simulink model "insulinGlucoseSimHumanCtrl_Harness1"  (R2019a)
settings: Solver=ode3  StartTime=0  StopTime=500  RelTol=1e-3  EnableMultiTasking=on
settings Model: Creator=yangy  LastModifiedBy=yangy
settings SolverCC: MaxConsecutiveZCs=100
settings DataIOCC: LimitDataPoints=on  SaveFormat=Array  SignalLoggingSaveFormat=ModelDataLogs  ReturnWorkspaceOutputs=off
settings OptimizationCC: ExpressionDepthLimit=2147483647  LifeSpan=inf
settings DebuggingCC: UnderspecifiedInitializationDetection=Classic  MergeDetectMultiDrivingBlocksExec=none  FcnCallInpInsideContextMsg=warning  StateNameClashWarn=warning  SFUnexpectedBacktrackingDiag=warning  SFNoUnconditionalDefaultTransitionDiag=warning  SFExecutionAtInitializationDiag=none  ArithmeticOperatorsInVariantConditions=warning
settings HardwareCC: ProdBitPerPointer=32  ProdBitPerSizeT=32  ProdBitPerPtrDiffT=32  ProdLargestAtomicFloat=None  ProdIntDivRoundTo=Undefined  ProdEndianess=Unspecified  ProdWordSize=32  ProdHWDeviceType=32-bit Generic
settings ModelReferenceCC: PropagateSignalLabelsOutOfModel=off
settings SFSimCC: SimUseLocalCustomCode=off  SimParseCustomCode=off
settings RTWCC: RTWUseLocalCustomCode=off
settings CodeAppCC: StateflowObjectComments=on
settings GRTTargetCC: TargetLangStandard=C89/C90 (ANSI)  GeneratePreprocessorConditionals=Disable all  CombineOutputUpdateFcns=off  GRTInterface=on
settings ConfigComp: CovMetricSettings=dw  CovHtmlReporting=on  CovSaveCumulativeToWorkspaceVar=on  CovSaveSingleToWorkspaceVar=on  CovExternalEMLEnable=off

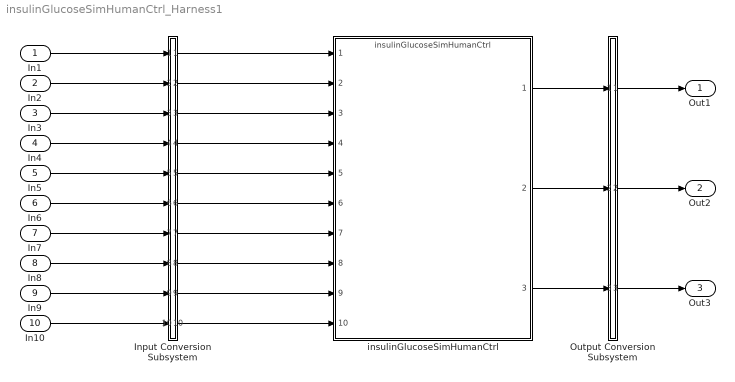
== system insulinGlucoseSimHumanCtrl_Harness1 ==
  In1 : Inport  OutDataTypeStr=double  PortDimensions=[1]  SampleTime=0
  In2 : Inport  Port=2  OutDataTypeStr=double  PortDimensions=[1]  SampleTime=0
  In3 : Inport  Port=3  OutDataTypeStr=double  PortDimensions=[1]  SampleTime=0
  In4 : Inport  Port=4  OutDataTypeStr=double  PortDimensions=[1]  SampleTime=0
  In5 : Inport  Port=5  OutDataTypeStr=double  PortDimensions=[1]  SampleTime=0
  In6 : Inport  Port=6  OutDataTypeStr=double  PortDimensions=[1]  SampleTime=0
  In7 : Inport  Port=7  OutDataTypeStr=double  PortDimensions=[1]  SampleTime=0
  In8 : Inport  Port=8  OutDataTypeStr=double  PortDimensions=[1]  SampleTime=0
  In9 : Inport  Port=9  OutDataTypeStr=double  PortDimensions=[1]  SampleTime=0
  In10 : Inport  Port=10  OutDataTypeStr=double  PortDimensions=[1]  SampleTime=0
  Input Conversion Subsystem : Subsystem  Tag=__SLT_ICS__  Description=|
      | Signal spec.
      | and routing
      settings: AttributesFormatString=%<Description>
  Output Conversion Subsystem : Subsystem  Tag=__SLT_OCS__  Description=|
      | Signal spec.
      | and routing
      settings: AttributesFormatString=%<Description>
  insulinGlucoseSimHumanCtrl : ModelReference  ModelNameDialog=insulinGlucoseSimHumanCtrl  SimulationMode=Normal  ModelReferenceVersion=1.334
  Out1 : Outport  OutDataTypeStr=double  PortDimensions=[1]
  Out2 : Outport  Port=2  OutDataTypeStr=double  PortDimensions=[1]
  Out3 : Outport  Port=3  OutDataTypeStr=double  PortDimensions=[1]
  wires:
  In1/1 -> Input Conversion Subsystem/1(Inport_1)
  In2/1 -> Input Conversion Subsystem/2(Inport_2)
  In3/1 -> Input Conversion Subsystem/3(Inport_3)
  In4/1 -> Input Conversion Subsystem/4(Inport_4)
  In5/1 -> Input Conversion Subsystem/5(Inport_5)
  In6/1 -> Input Conversion Subsystem/6(Inport_6)
  In7/1 -> Input Conversion Subsystem/7(Inport_7)
  In8/1 -> Input Conversion Subsystem/8(Inport_8)
  In9/1 -> Input Conversion Subsystem/9(Inport_9)
  In10/1 -> Input Conversion Subsystem/10(Inport_10)
  Output Conversion Subsystem/1(Outport_1) -> Out1/1
  Output Conversion Subsystem/2(Outport_2) -> Out2/1
  Output Conversion Subsystem/3(Outport_3) -> Out3/1
  Input Conversion Subsystem/1(Outport_1) -> insulinGlucoseSimHumanCtrl/1
  Input Conversion Subsystem/2(Outport_2) -> insulinGlucoseSimHumanCtrl/2
  Input Conversion Subsystem/3(Outport_3) -> insulinGlucoseSimHumanCtrl/3
  Input Conversion Subsystem/4(Outport_4) -> insulinGlucoseSimHumanCtrl/4
  Input Conversion Subsystem/5(Outport_5) -> insulinGlucoseSimHumanCtrl/5
  Input Conversion Subsystem/6(Outport_6) -> insulinGlucoseSimHumanCtrl/6
  Input Conversion Subsystem/7(Outport_7) -> insulinGlucoseSimHumanCtrl/7
  Input Conversion Subsystem/8(Outport_8) -> insulinGlucoseSimHumanCtrl/8
  Input Conversion Subsystem/9(Outport_9) -> insulinGlucoseSimHumanCtrl/9
  Input Conversion Subsystem/10(Outport_10) -> insulinGlucoseSimHumanCtrl/10
  insulinGlucoseSimHumanCtrl/1 -> Output Conversion Subsystem/1(Inport_1)
  insulinGlucoseSimHumanCtrl/2 -> Output Conversion Subsystem/2(Inport_2)
  insulinGlucoseSimHumanCtrl/3 -> Output Conversion Subsystem/3(Inport_3)

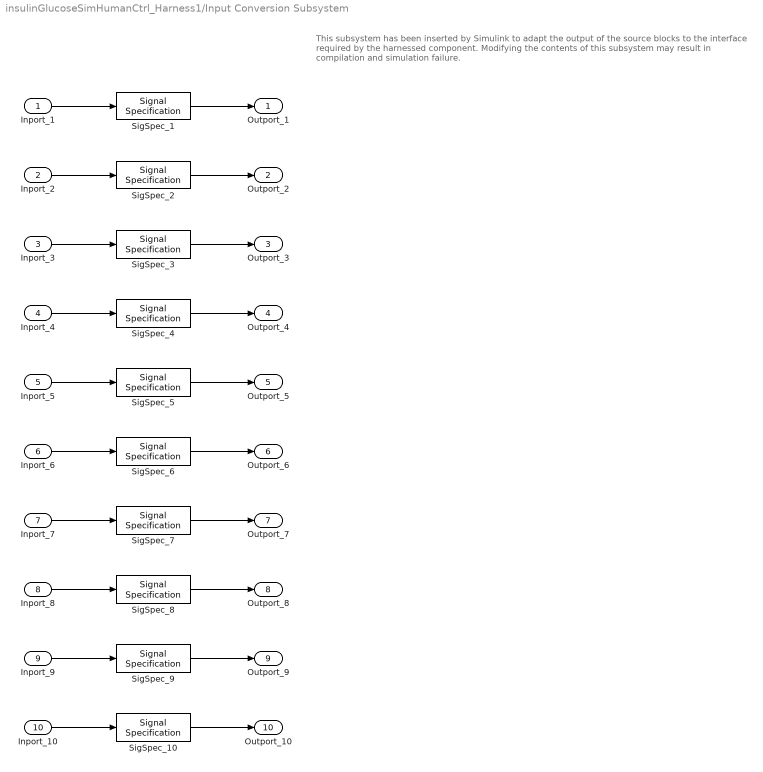
== system insulinGlucoseSimHumanCtrl_Harness1/Input Conversion Subsystem ==
  note: This subsystem has been inserted by Simulink to adapt the output of the source blocks to the interface required by the harnessed component.
      |  Modifying the contents of this subsystem may result in compilation and simulation failure.
  Inport_1 : Inport
  Inport_2 : Inport  Port=2
  Inport_3 : Inport  Port=3
  Inport_4 : Inport  Port=4
  Inport_5 : Inport  Port=5
  Inport_6 : Inport  Port=6
  Inport_7 : Inport  Port=7
  Inport_8 : Inport  Port=8
  Inport_9 : Inport  Port=9
  Inport_10 : Inport  Port=10
  SigSpec_{1..10} (10 alike) : SignalSpecification  OutDataTypeStr=double  Dimensions=[1]  SampleTime=[0, 0]
  Outport_1 : Outport
  Outport_2 : Outport  Port=2
  Outport_3 : Outport  Port=3
  Outport_4 : Outport  Port=4
  Outport_5 : Outport  Port=5
  Outport_6 : Outport  Port=6
  Outport_7 : Outport  Port=7
  Outport_8 : Outport  Port=8
  Outport_9 : Outport  Port=9
  Outport_10 : Outport  Port=10
  wires:
  SigSpec_1/1 -> Outport_1/1
  Inport_1/1 -> SigSpec_1/1
  SigSpec_2/1 -> Outport_2/1
  Inport_2/1 -> SigSpec_2/1
  SigSpec_3/1 -> Outport_3/1
  Inport_3/1 -> SigSpec_3/1
  SigSpec_4/1 -> Outport_4/1
  Inport_4/1 -> SigSpec_4/1
  SigSpec_5/1 -> Outport_5/1
  Inport_5/1 -> SigSpec_5/1
  SigSpec_6/1 -> Outport_6/1
  Inport_6/1 -> SigSpec_6/1
  SigSpec_7/1 -> Outport_7/1
  Inport_7/1 -> SigSpec_7/1
  SigSpec_8/1 -> Outport_8/1
  Inport_8/1 -> SigSpec_8/1
  SigSpec_9/1 -> Outport_9/1
  Inport_9/1 -> SigSpec_9/1
  SigSpec_10/1 -> Outport_10/1
  Inport_10/1 -> SigSpec_10/1

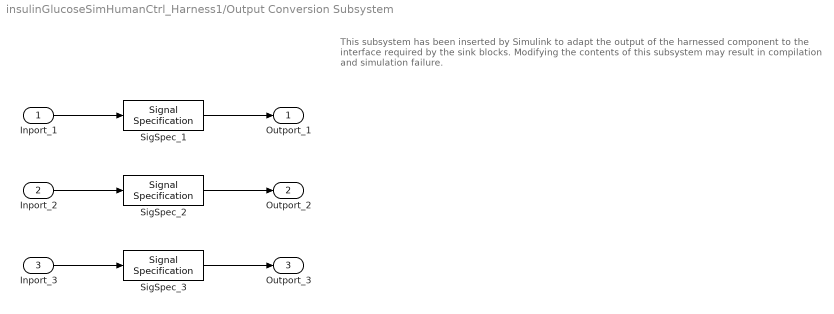
== system insulinGlucoseSimHumanCtrl_Harness1/Output Conversion Subsystem ==
  note: This subsystem has been inserted by Simulink to adapt the output of the harnessed component to the interface required by the sink blocks.
      |  Modifying the contents of this subsystem may result in compilation and simulation failure.
  Inport_1 : Inport
  Inport_2 : Inport  Port=2
  Inport_3 : Inport  Port=3
  SigSpec_1 : SignalSpecification  OutDataTypeStr=double  Dimensions=[1]
  SigSpec_2 : SignalSpecification  OutDataTypeStr=double  Dimensions=[1]
  SigSpec_3 : SignalSpecification  OutDataTypeStr=double  Dimensions=[1]
  Outport_1 : Outport
  Outport_2 : Outport  Port=2
  Outport_3 : Outport  Port=3
  wires:
  Inport_1/1 -> SigSpec_1/1
  SigSpec_1/1 -> Outport_1/1
  Inport_2/1 -> SigSpec_2/1
  SigSpec_2/1 -> Outport_2/1
  Inport_3/1 -> SigSpec_3/1
  SigSpec_3/1 -> Outport_3/1
